simulink model "gm_iopid"  (R2021b)
settings: Solver=FixedStepDiscrete  StartTime=0.0  StopTime=100e-3  RelTol=1e-3
libraries: hdlmdlgenlib x1
Description:
  | Symmetric FIR Filter
  | This example shows how to use HDL Coder(TM) to check, generate,
  | and verify HDL for a fixed-point symmetric FIR filter.
settings Model: Creator=The MathWorks, Inc.  LastModifiedBy=Marco Milanesi
settings SolverCC: AlgebraicLoopSolver=TrustRegion  AutoInsertRateTranBlk=on
settings DataIOCC: LimitDataPoints=on  SaveFormat=Array  SaveOutput=off  SignalLogging=off  SaveTime=off  ReturnWorkspaceOutputs=off  SignalLoggingName=logsOut
settings OptimizationCC: BlockReduction=off  BooleanDataType=off  ConditionallyExecuteInputs=off  DefaultParameterBehavior=Inlined  InheritOutputTypeSmallerThanSingle=on  InlineInvariantSignals=on  ExpressionDepthLimit=2147483647  InitFltsAndDblsToZero=on  LifeSpan=inf  BufferReusableBoundary=off
settings DebuggingCC: AlgebraicLoopMsg=error  SaveWithParameterizedLinksMsg=none  UnderspecifiedInitializationDetection=Classic  MergeDetectMultiDrivingBlocksExec=none  CheckExecutionContextPreStartOutputMsg=on  SignalResolutionControl=TryResolveAllWithWarning  InheritedTsInSrcMsg=none  MultiTaskDSMMsg=warning  MultiTaskCondExecSysMsg=none  SingleTaskRateTransMsg=error  IntegerOverflowMsg=none  ParameterPrecisionLossMsg=none  FcnCallInpInsideContextMsg=warning  BusObjectLabelMismatch=none  StateNameClashWarn=warning  SFUnexpectedBacktrackingDiag=warning  SFNoUnconditionalDefaultTransitionDiag=warning  SFExecutionAtInitializationDiag=none  SFMachineParentedDataDiag=warning  IntegerSaturationMsg=none  ArithmeticOperatorsInVariantConditions=warning
settings HardwareCC: ProdBitPerPointer=32  ProdBitPerSizeT=32  ProdBitPerPtrDiffT=32  ProdLargestAtomicFloat=None  ProdIntDivRoundTo=Undefined  ProdEndianess=Unspecified  ProdWordSize=32  ProdHWDeviceType=ASIC/FPGA  TargetUnknown=on  ProdEqTarget=off
settings ModelReferenceCC: PropagateSignalLabelsOutOfModel=off
settings SFSimCC: SimUseLocalCustomCode=off  CustomCodeUndefinedFunction=UseInterfaceOnly
settings RTWCC: RTWUseLocalCustomCode=off
settings CodeAppCC: StateflowObjectComments=on
settings GRTTargetCC: TargetFcnLib=ansi_tfl_tmw.mat  TargetLangStandard=C89/C90 (ANSI)  CombineOutputUpdateFcns=off  GRTInterface=on
settings ConfigComp: CovMetricSettings=dw  CovSaveCumulativeToWorkspaceVar=on  CovSaveSingleToWorkspaceVar=on  CovExternalEMLEnable=off

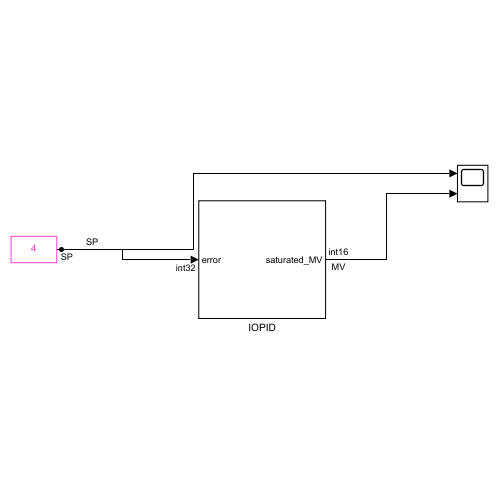
[thumbnail: Simulink's stored preview of the top-level diagram]
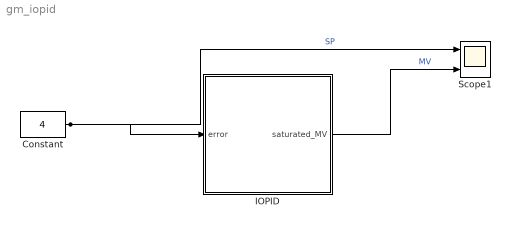
== system gm_iopid ==
  Constant : Constant  Value=4  OutDataTypeStr=fixdt(1,32,0)
  IOPID : Subsystem
  Scope1 : Scope  NumInputPorts=2
  wires:
  IOPID/1(saturated_MV) -> Scope1/2  "MV"
  Constant/1 -> IOPID/1(error), Scope1/1  "SP"

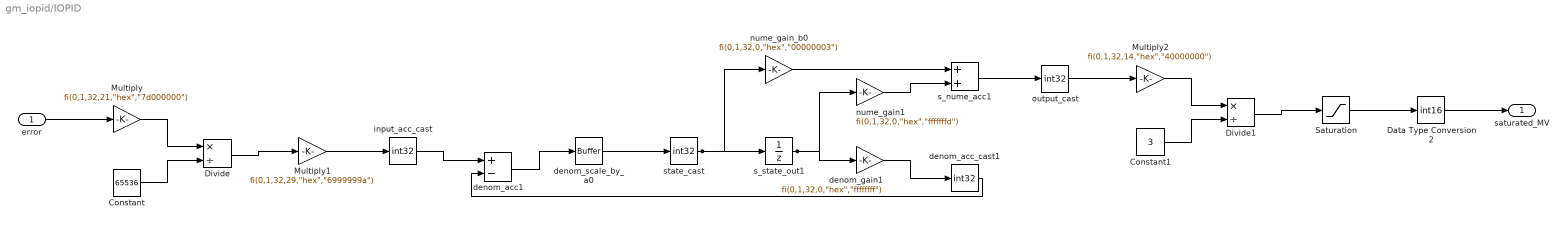
== system gm_iopid/IOPID ==
  error : Inport  OutDataTypeStr=int32  PortDimensions=1  SampleTime=8e-08
  Constant : Constant  Value=65536  OutDataTypeStr=int32
  Constant1 : Constant  Value=3  OutDataTypeStr=int32
  Data Type Conversion2 : DataTypeConversion  OutDataTypeStr=int16  SampleTime=8e-08
  Divide : Product  Inputs=*/  OutDataTypeStr=int32  RndMeth=Zero  SaturateOnIntegerOverflow=on  SampleTime=8e-08
  Divide1 : Product  Inputs=*/  OutDataTypeStr=int32  RndMeth=Zero  SaturateOnIntegerOverflow=on  SampleTime=8e-08
  Multiply : Gain  Gain="fi(0,1,32,21,\"hex\",\"7d000000\")"  ParamDataTypeStr=fixdt(1, 32, 21)  OutDataTypeStr=int32  SampleTime=8e-08
  Multiply1 : Gain  Gain="fi(0,1,32,29,\"hex\",\"6999999a\")"  ParamDataTypeStr=fixdt(1, 32, 29)  OutDataTypeStr=int32  SampleTime=8e-08
  Multiply2 : Gain  Gain="fi(0,1,32,14,\"hex\",\"40000000\")"  ParamDataTypeStr=fixdt(1, 32, 14)  OutDataTypeStr=int32  SampleTime=8e-08
  Saturation : Saturate  UpperLimit="fi(0,1,32,0,\"hex\",\"000000ff\")"  LowerLimit="fi(0,1,32,0,\"hex\",\"00000000\")"  SampleTime=8e-08  OutDataTypeStr=int32
  denom_acc1 : Sum  Inputs=+-  AccumDataTypeStr=int32  OutDataTypeStr=int32  SampleTime=8e-08
  denom_acc_cast1 : DataTypeConversion  OutDataTypeStr=int32  SampleTime=8e-08
  denom_gain1 : Gain  Gain="fi(0,1,32,0,\"hex\",\"ffffffff\")"  ParamDataTypeStr=fixdt(1, 32, 0)  OutDataTypeStr=int32  SampleTime=8e-08
  denom_scale_by_a0 : hdlmdlgenlib/Buffer
      settings: SourceProductBaseCode=SL
  input_acc_cast : DataTypeConversion  OutDataTypeStr=int32  SampleTime=8e-08
  nume_gain1 : Gain  Gain="fi(0,1,32,0,\"hex\",\"fffffffd\")"  ParamDataTypeStr=fixdt(1, 32, 0)  OutDataTypeStr=int32  SampleTime=8e-08
  nume_gain_b0 : Gain  Gain="fi(0,1,32,0,\"hex\",\"00000003\")"  ParamDataTypeStr=fixdt(1, 32, 0)  OutDataTypeStr=int32  SampleTime=8e-08
  output_cast : DataTypeConversion  OutDataTypeStr=int32  SampleTime=8e-08
  s_nume_acc1 : Sum  OutDataTypeStr=int32  SampleTime=8e-08
  s_state_out1 : UnitDelay  InitialCondition="fi(0,1,32,0,\"hex\",\"00000000\")"  SampleTime=8e-08
  state_cast : DataTypeConversion  OutDataTypeStr=int32  SampleTime=8e-08
  saturated_MV : Outport  OutDataTypeStr=fixdt(1,16,0)  SampleTime=8e-08  VectorParamsAs1DForOutWhenUnconnected=off
  wires:
  error/1 -> Multiply/1
  Constant/1 -> Divide/2
  Constant1/1 -> Divide1/2
  Data Type Conversion2/1 -> saturated_MV/1
  Divide/1 -> Multiply1/1
  Divide1/1 -> Saturation/1
  Multiply/1 -> Divide/1
  Multiply1/1 -> input_acc_cast/1
  Multiply2/1 -> Divide1/1
  Saturation/1 -> Data Type Conversion2/1
  input_acc_cast/1 -> denom_acc1/1
  denom_acc_cast1/1 -> denom_acc1/2
  denom_acc1/1 -> denom_scale_by_a0/1
  denom_scale_by_a0/1 -> state_cast/1
  state_cast/1 -> nume_gain_b0/1, s_state_out1/1
  s_state_out1/1 -> nume_gain1/1, denom_gain1/1
  denom_gain1/1 -> denom_acc_cast1/1
  nume_gain_b0/1 -> s_nume_acc1/1
  nume_gain1/1 -> s_nume_acc1/2
  s_nume_acc1/1 -> output_cast/1
  output_cast/1 -> Multiply2/1
